simulink model "motor_identification"  (R2023a)
settings: Solver=VariableStepAuto  StartTime=0.0  StopTime=inf  FixedStep=0.01  RelTol=1e-3
libraries: instrumentseriallib x3, eeDiscretePi x2, slpidlib x2, svdutilitieslib x1, etargetslib x1
settings Model: Creator=arian  LastModifiedBy=arian
settings DebuggingCC: ParameterOverflowMsg=none  ParameterPrecisionLossMsg=none
settings HardwareCC: ProdBitPerLong=64  ProdHWDeviceType=Intel->x86-64 (Linux 64)
settings RTWCC: Description=Simulink Desktop Real-Time  SystemTargetFile=sldrt.tlc  TemplateMakefile=sldrt.tmf  RTWCompilerOptimization=on
settings CodeAppCC: MaxIdLength=95
settings SimulinkDesktopRealTimeCC: TargetLibSuffix=_sldrt.a  TargetPreCompLibLocation=C:\Program Files\MATLAB\R2023a\toolbox\sldrt\lib\win64

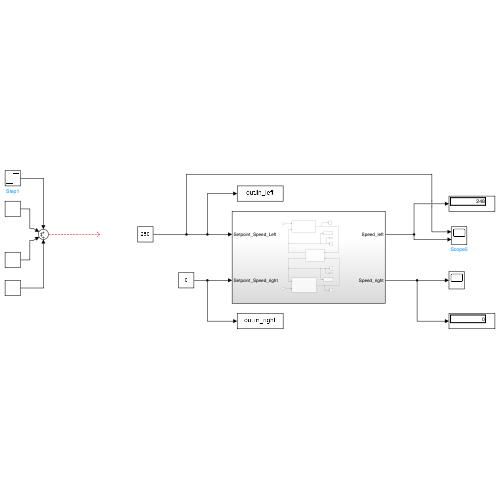
[thumbnail: Simulink's stored preview of the top-level diagram]
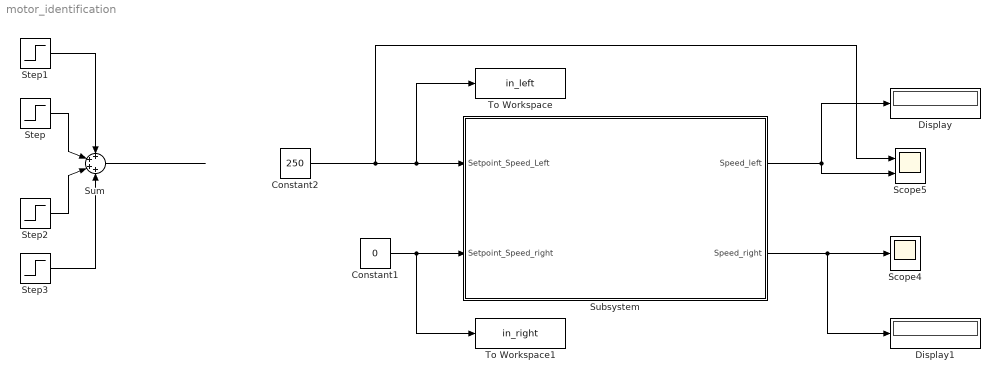
== system motor_identification ==
  Constant1 : Constant  Value=0  OutDataTypeStr=uint8
  Constant2 : Constant  Value=250  OutDataTypeStr=uint8
  Display : Display
  Display1 : Display
  Scope4 : Scope
  Scope5 : Scope  NumInputPorts=2
  Step : Step  Time=0  After=50  SampleTime=0
  Step1 : Step  Time=5  After=50  SampleTime=0
  Step2 : Step  Time=10  After=50  SampleTime=0
  Step3 : Step  Time=15  After=50  SampleTime=0
  Subsystem : Subsystem
  Sum : Sum  Inputs=++++
  To Workspace : ToWorkspace  VariableName=in_left  SaveFormat=Timeseries  SampleTime=-1
  To Workspace1 : ToWorkspace  VariableName=in_right  SaveFormat=Timeseries  SampleTime=-1
  wires:
  Sum/1 -> ?
  Constant1/1 -> To Workspace1/1, Subsystem/2(Setpoint_Speed_right)
  Subsystem/1(Speed_left) -> Scope5/2, Display/1
  Subsystem/2(Speed_right) -> Display1/1, Scope4/1
  Step/1 -> Sum/2
  Step2/1 -> Sum/3
  Step1/1 -> Sum/1
  Step3/1 -> Sum/4
  Constant2/1 -> Scope5/1, Subsystem/1(Setpoint_Speed_Left), To Workspace/1

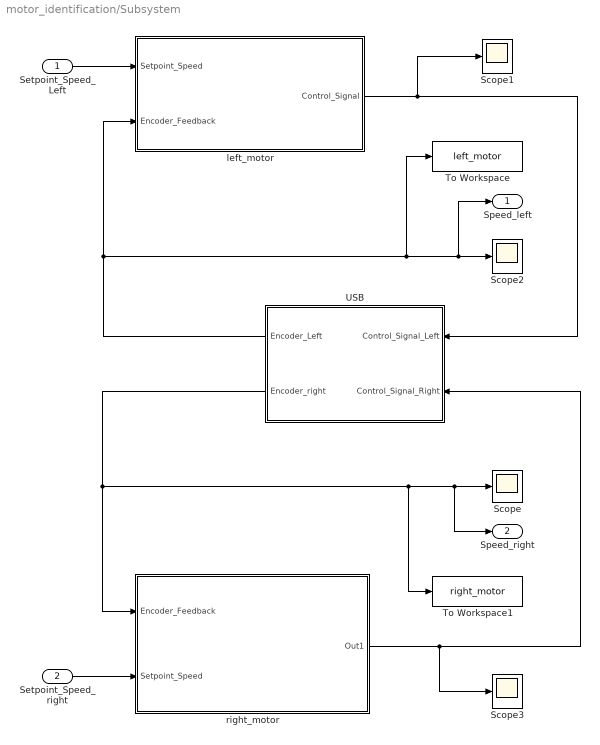
== system motor_identification/Subsystem ==
  Setpoint_Speed_Left : Inport
  Setpoint_Speed_right : Inport  Port=2
  Scope{,1..3} (4 alike) : Scope
  To Workspace : ToWorkspace  VariableName=left_motor  SampleTime=-1
  To Workspace1 : ToWorkspace  VariableName=right_motor  SampleTime=-1
  USB : Subsystem
  left_motor : Subsystem
  right_motor : Subsystem
  Speed_left : Outport
  Speed_right : Outport  Port=2
  wires:
  left_motor/1(Control_Signal) -> Scope1/1, USB/1(Control_Signal_Left)
  Setpoint_Speed_Left/1 -> left_motor/1(Setpoint_Speed)
  right_motor/1(Out1) -> Scope3/1, USB/2(Control_Signal_Right)
  USB/2(Encoder_right) -> right_motor/1(Encoder_Feedback), Speed_right/1, Scope/1, To Workspace1/1
  USB/1(Encoder_Left) -> Speed_left/1, Scope2/1, To Workspace/1, left_motor/2(Encoder_Feedback)
  Setpoint_Speed_right/1 -> right_motor/2(Setpoint_Speed)

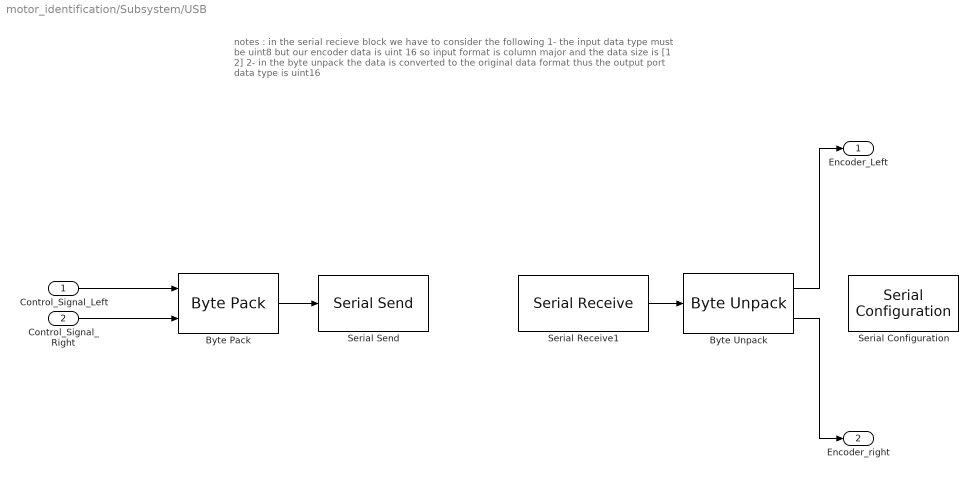
== system motor_identification/Subsystem/USB ==
  note: notes :
      | in the serial recieve block we have to consider the following
      | 1- the input data type must be uint8 but our encoder data is uint 16 so input format is column major and the data size is [1 2]
      | 2- in the byte unpack the data is converted to the original data format thus the output port data type is uint16
  Control_Signal_Left : Inport
  Control_Signal_Right : Inport  Port=2
  Byte Pack : svdutilitieslib/Byte Pack  maskPackedDataType=uint8  datatypes={'uint8';'uint8'}  byteAlign=1  blockPlatform=arduinoert
  Byte Unpack : etargetslib/Byte Unpack  dimensions={[1],[1]}  datatypes={'uint16','uint16'}  byteAlign=1
      settings: LibrarySourceBlock=embeddedtargetslib/Host Communication/Byte Unpack
  Serial Configuration : instrumentseriallib/Serial Configuration  Priority=-200000  PortSel=COM10  Port=COM10  ComPort=COM10  BaudRate=115200  DataBits=8  Parity=none  StopBits=1  ByteOrder=little-endian  FlowControl=none  Timeout=10  SimulateUsing=Interpreted execution  BlockInModel=on  aMode=1
      settings: LibrarySourceBlock=embeddedtargetslib/Host Communication/Serial Configuration
  Serial Receive1 : instrumentseriallib/Serial Receive  Priority=1  PortSel=COM10  Port=COM10  ComPort=COM10  DataType=uint8  SaveDataType=uint8  ToggleHeader=off  Header=[]  ToggleTerminator=off  Terminator=<none>  CustomTerminator=[]  InputFormat=Column major  ToggleDataSize=on  DataSize=[2 2]  EnableBlockingMode=on  ActionDataUnavailable=Output last received value  ActionWhenDataUnavailable=Output last received value  CustomValue=0  SampleTime=0.01  SimulateUsing=Interpreted execution  BlockInModel=on  aMode=1
  Serial Send : instrumentseriallib/Serial Send  Priority=1  PortSel=COM10  Port=COM10  ComPort=COM10  Header=[]  Terminator=<none>  CustomTerminator=[]  EnableBlockingMode=on  SimulateUsing=Interpreted execution  BlockInModel=on  aMode=1
      settings: LibrarySourceBlock=embeddedtargetslib/Host Communication/Serial Send
  Encoder_Left : Outport
  Encoder_right : Outport  Port=2
  wires:
  Serial Receive1/1 -> Byte Unpack/1
  Byte Unpack/2 -> Encoder_right/1
  Byte Unpack/1 -> Encoder_Left/1
  Byte Pack/1 -> Serial Send/1
  Control_Signal_Right/1 -> Byte Pack/2
  Control_Signal_Left/1 -> Byte Pack/1

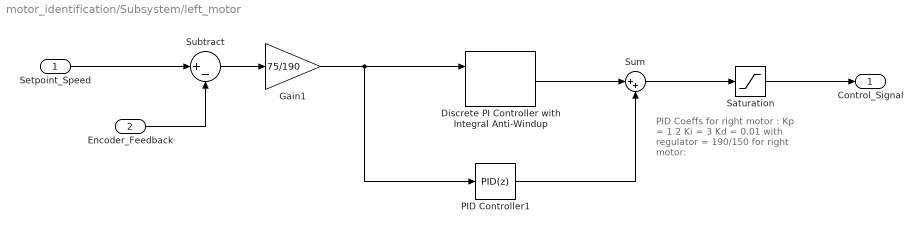
== system motor_identification/Subsystem/left_motor ==
  note: PID Coeffs
      |
      | for right motor :
      | Kp = 1.2
      | Ki = 3
      | Kd = 0.01
      | with regulator = 190/150
      |
      | for right motor:
  Setpoint_Speed : Inport
  Encoder_Feedback : Inport  Port=2
  Discrete PI Controller with Integral Anti-Windup : eeDiscretePi/Discrete PI Controller with Integral Anti-Windup  Kp=1.2  Ki=3  x0=0  B=100  A=0  Ts=-1
      settings: LibrarySourceBlock=|
      | ee_sl_lib/General Control/Discrete PI Controller
      | with Integral Anti-Windup
  Gain1 : Gain  Gain=75/190  OutDataTypeStr=int32
  PID Controller1 : slpidlib/PID Controller  Controller=PID  Form=Parallel  TimeDomain=Discrete-time  UseExternalTs=off  SampleTime=-1  IntegratorMethod=Forward Euler  FilterMethod=Forward Euler  ControllerParametersSource=internal  P=0  I=0  UseKiTs=off  D=0.01  N=20  UseFilter=on  TunerSelectOption=Transfer Function Based (PID Tuner App)  InitialConditionSource=internal  InitialConditionForIntegrator=0  InitialConditionForFilter=0  DifferentiatorICPrevScaledInput=0  ExternalReset=none  TrackingMode=off  Kt=1  LimitOutput=off  SatLimitsSource=internal  UpperSaturationLimit=inf  LowerSaturationLimit=-inf  LinearizeAsGain=on  AntiWindupMode=none  Kb=1  LimitIntegrator=off  UpperIntegratorSaturationLimit=inf  LowerIntegratorSaturationLimit=-inf  RndMeth=Round  PGainOutDataTypeStr=int32  PProdOutDataTypeStr=int32  POutMin=[]  POutMax=[]  IGainOutDataTypeStr=int32  IProdOutDataTypeStr=int32  IOutMin=[]  IOutMax=[]  DGainOutDataTypeStr=int32  DProdOutDataTypeStr=int32  DOutMin=[]  DOutMax=[]  NGainOutDataTypeStr=int32  NProdOutDataTypeStr=int32  NOutMin=[]  NOutMax=[]  SumOutDataTypeStr=int32  SumOutMin=[]  SumOutMax=[]  SaturationOutMin=[]  SaturationOutMax=[]  PParamMin=[]  PParamMax=[]  IParamMin=[]  IParamMax=[]  DParamMin=[]  DParamMax=[]  NParamMin=[]  NParamMax=[]  KbParamMin=[]  KbParamMax=[]  KtParamMin=[]  KtParamMax=[]  KbOutMin=[]  KbOutMax=[]  KtOutMin=[]  KtOutMax=[]  IntegratorOutMin=[]  IntegratorOutMax=[]  FilterOutMin=[]  FilterOutMax=[]  SumI1OutMin=[]  SumI1OutMax=[]  SumI2OutMin=[]  SumI2OutMax=[]  SumI3OutMin=[]  SumI3OutMax=[]  SumI4OutMin=[]  SumI4OutMax=[]  SumDOutMin=[]  SumDOutMax=[]  DifferentiatorOutMin=[]  DifferentiatorOutMax=[]  FilterDiffOutCoefMin=[]  FilterDiffOutCoefMax=[]  ReciprocalOutMin=[]  ReciprocalOutMax=[]  SumDenOutMin=[]  SumDenOutMax=[]  SumNumOutMin=[]  SumNumOutMax=[]  DivideOutMin=[]  DivideOutMax=[]  UdiffTsProdOutMin=[]  UdiffTsProdOutMax=[]  NTsProdOutMin=[]  NTsProdOutMax=[]  UintegralTsProdOutMin=[]  UintegralTsProdOutMax=[]  UngainTsProdOutMin=[]  UngainTsProdOutMax=[]  ClampingZeroOutDataTypeStr=Inherit: Inherit via back propagation  ClampingZeroOutMin=[]  ClampingZeroOutMax=[]  FilterDenConstantOutDataTypeStr=Inherit: Inherit via back propagation  FilterDenConstantOutMin=[]  FilterDenConstantOutMax=[]  PCopyOutDataTypeStr=Inherit: Inherit via back propagation  PCopyOutMin=[]  PCopyOutMax=[]  NCopyOutDataTypeStr=Inherit: Inherit via back propagation  NCopyOutMin=[]  NCopyOutMax=[]  IntegratorContinuousStateAttributes=''  IntegratorStateMustResolveToSignalObject=off  IntegratorRTWStateStorageClass=Auto  FilterContinuousStateAttributes=''  FilterStateMustResolveToSignalObject=off  FilterRTWStateStorageClass=Auto  ParallelPVariant=InternalParameters  IdealPVariant=Disabled  IVariant=InternalParameters  DVariant=InternalParameters  IntegratorVariant=Discrete  SatVariant=Disabled  AWVariant=Passthrough  PCopyVariant=Disabled  TRVariant=Disabled  FdbkBlocksVariant=Forward  IdealPFdbkVariant=Disabled  SatFdbkVariant=Disabled  DerivativeFilterVariant=ForwardEulerFilter  NVariant=InternalParameters  NCopyVariant=Disabled  FilterICVariant=InternalICsFilter  IntegratorICVariant=InternalICs  ExternalResetVariant=Disabled  TRSumVariant=Passthrough  SumFdbkVariant=Disabled  SumVariant=Sum_PID  TsampFilterVariant=InternalTs  TsampNgainVariant=Passthrough  TsampIntegralVariant=Disabled_SignalSpec  ExternalSaturationOutDataTypeStr=Inherit: Same as second input
  Saturation : Saturate  UpperLimit=100  LowerLimit=0  OutDataTypeStr=uint8
  Subtract : Sum  Inputs=|+-  OutDataTypeStr=int32  RndMeth=Round
  Sum : Sum  Inputs=|++
  Control_Signal : Outport
  wires:
  Setpoint_Speed/1 -> Subtract/1
  PID Controller1/1 -> Sum/2
  Gain1/1 -> PID Controller1/1, Discrete PI Controller with Integral Anti-Windup/1
  Sum/1 -> Saturation/1
  Subtract/1 -> Gain1/1
  Discrete PI Controller with Integral Anti-Windup/1 -> Sum/1
  Encoder_Feedback/1 -> Subtract/2
  Saturation/1 -> Control_Signal/1

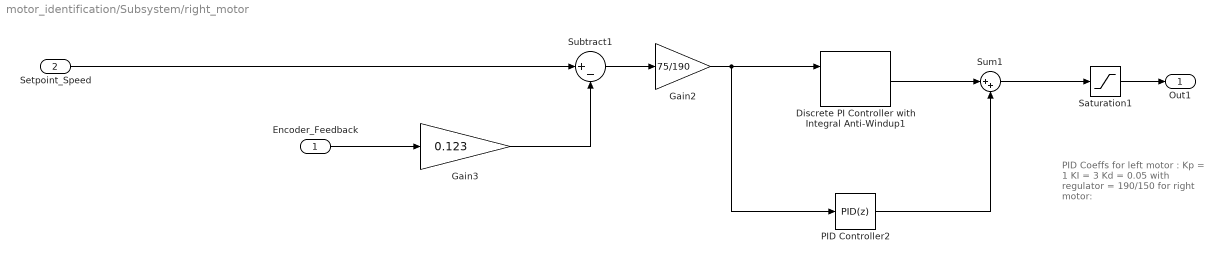
== system motor_identification/Subsystem/right_motor ==
  note: PID Coeffs
      |
      | for left motor :
      | Kp = 1
      | KI = 3
      | Kd = 0.05
      | with regulator = 190/150
      |
      | for right motor:
  Encoder_Feedback : Inport
  Setpoint_Speed : Inport  Port=2
  Discrete PI Controller with Integral Anti-Windup1 : eeDiscretePi/Discrete PI Controller with Integral Anti-Windup  Kp=1  Ki=3  x0=0  B=100  A=0  Ts=-1
      settings: LibrarySourceBlock=|
      | ee_sl_lib/General Control/Discrete PI Controller
      | with Integral Anti-Windup
  Gain2 : Gain  Gain=75/190  OutDataTypeStr=int32
  Gain3 : Gain  Gain=0.123  OutDataTypeStr=int32
  PID Controller2 : slpidlib/PID Controller  Controller=PID  Form=Parallel  TimeDomain=Discrete-time  UseExternalTs=off  SampleTime=-1  IntegratorMethod=Forward Euler  FilterMethod=Forward Euler  ControllerParametersSource=internal  P=0  I=0  UseKiTs=off  D=0.05  N=20  UseFilter=on  TunerSelectOption=Transfer Function Based (PID Tuner App)  InitialConditionSource=internal  InitialConditionForIntegrator=0  InitialConditionForFilter=0  DifferentiatorICPrevScaledInput=0  ExternalReset=none  TrackingMode=off  Kt=1  LimitOutput=off  SatLimitsSource=internal  UpperSaturationLimit=inf  LowerSaturationLimit=-inf  LinearizeAsGain=on  AntiWindupMode=none  Kb=1  LimitIntegrator=off  UpperIntegratorSaturationLimit=inf  LowerIntegratorSaturationLimit=-inf  RndMeth=Round  PGainOutDataTypeStr=int32  PProdOutDataTypeStr=int32  POutMin=[]  POutMax=[]  IGainOutDataTypeStr=int32  IProdOutDataTypeStr=int32  IOutMin=[]  IOutMax=[]  DGainOutDataTypeStr=int32  DProdOutDataTypeStr=int32  DOutMin=[]  DOutMax=[]  NGainOutDataTypeStr=int32  NProdOutDataTypeStr=int32  NOutMin=[]  NOutMax=[]  SumOutDataTypeStr=int32  SumOutMin=[]  SumOutMax=[]  SaturationOutMin=[]  SaturationOutMax=[]  PParamMin=[]  PParamMax=[]  IParamMin=[]  IParamMax=[]  DParamMin=[]  DParamMax=[]  NParamMin=[]  NParamMax=[]  KbParamMin=[]  KbParamMax=[]  KtParamMin=[]  KtParamMax=[]  KbOutMin=[]  KbOutMax=[]  KtOutMin=[]  KtOutMax=[]  IntegratorOutMin=[]  IntegratorOutMax=[]  FilterOutMin=[]  FilterOutMax=[]  SumI1OutMin=[]  SumI1OutMax=[]  SumI2OutMin=[]  SumI2OutMax=[]  SumI3OutMin=[]  SumI3OutMax=[]  SumI4OutMin=[]  SumI4OutMax=[]  SumDOutMin=[]  SumDOutMax=[]  DifferentiatorOutMin=[]  DifferentiatorOutMax=[]  FilterDiffOutCoefMin=[]  FilterDiffOutCoefMax=[]  ReciprocalOutMin=[]  ReciprocalOutMax=[]  SumDenOutMin=[]  SumDenOutMax=[]  SumNumOutMin=[]  SumNumOutMax=[]  DivideOutMin=[]  DivideOutMax=[]  UdiffTsProdOutMin=[]  UdiffTsProdOutMax=[]  NTsProdOutMin=[]  NTsProdOutMax=[]  UintegralTsProdOutMin=[]  UintegralTsProdOutMax=[]  UngainTsProdOutMin=[]  UngainTsProdOutMax=[]  ClampingZeroOutDataTypeStr=Inherit: Inherit via back propagation  ClampingZeroOutMin=[]  ClampingZeroOutMax=[]  FilterDenConstantOutDataTypeStr=Inherit: Inherit via back propagation  FilterDenConstantOutMin=[]  FilterDenConstantOutMax=[]  PCopyOutDataTypeStr=Inherit: Inherit via back propagation  PCopyOutMin=[]  PCopyOutMax=[]  NCopyOutDataTypeStr=Inherit: Inherit via back propagation  NCopyOutMin=[]  NCopyOutMax=[]  IntegratorContinuousStateAttributes=''  IntegratorStateMustResolveToSignalObject=off  IntegratorRTWStateStorageClass=Auto  FilterContinuousStateAttributes=''  FilterStateMustResolveToSignalObject=off  FilterRTWStateStorageClass=Auto  ParallelPVariant=InternalParameters  IdealPVariant=Disabled  IVariant=InternalParameters  DVariant=InternalParameters  IntegratorVariant=Discrete  SatVariant=Disabled  AWVariant=Passthrough  PCopyVariant=Disabled  TRVariant=Disabled  FdbkBlocksVariant=Forward  IdealPFdbkVariant=Disabled  SatFdbkVariant=Disabled  DerivativeFilterVariant=ForwardEulerFilter  NVariant=InternalParameters  NCopyVariant=Disabled  FilterICVariant=InternalICsFilter  IntegratorICVariant=InternalICs  ExternalResetVariant=Disabled  TRSumVariant=Passthrough  SumFdbkVariant=Disabled  SumVariant=Sum_PID  TsampFilterVariant=InternalTs  TsampNgainVariant=Passthrough  TsampIntegralVariant=Disabled_SignalSpec  ExternalSaturationOutDataTypeStr=Inherit: Same as second input
  Saturation1 : Saturate  UpperLimit=100  LowerLimit=0  OutDataTypeStr=uint8
  Subtract1 : Sum  Inputs=|+-  OutDataTypeStr=int32  RndMeth=Round
  Sum1 : Sum  Inputs=|++
  Out1 : Outport
  wires:
  Discrete PI Controller with Integral Anti-Windup1/1 -> Sum1/1
  PID Controller2/1 -> Sum1/2
  Gain2/1 -> PID Controller2/1, Discrete PI Controller with Integral Anti-Windup1/1
  Subtract1/1 -> Gain2/1
  Sum1/1 -> Saturation1/1
  Setpoint_Speed/1 -> Subtract1/1
  Gain3/1 -> Subtract1/2
  Encoder_Feedback/1 -> Gain3/1
  Saturation1/1 -> Out1/1
